simulink model "gg_plus_lc_platoon"  (R2019a)
settings: Solver=ode23t  StartTime=0.0  StopTime=70  FixedStep=0.1  MaxStep=0.01  RelTol=1e-3
InitFcn:
  | load vehStatesBus
libraries: simulink x120, powerlib_meascontrol x14, dspsigops x7, autolibshared x7
(part 5 of 7)

== system gg_plus_lc_platoon/p3/Virtual Vehicle Following ==
  ego : Inport
  virtualLeader : Inport  Port=2
  leaderChange : Inport  Port=3
  extraSpaceFlag : Inport  Port=4
  Enable : EnablePort
  Bus Selector : BusSelector  OutputSignals=X,Xdot,u
  Bus Selector1 : BusSelector  OutputSignals=X,Xdot
  Chart : Stateflow chart  BlockKeywords=__PRM__SERIALIZED__DATA__:Stateflow Chart,Stateflow Diagram  TreatAsAtomicUnit=on
  Compare To Constant : simulink/Logic and Bit Operations/Compare To Constant  relop=>  const=0  OutDataTypeStr=boolean
  Compare To Constant1 : simulink/Logic and Bit Operations/Compare To Constant  relop=<  const=2*maxHeadwayError  OutDataTypeStr=boolean
  Compute Errors : Subsystem
  Mux : Mux  Inputs=2
  Scope : Scope  NumInputPorts=2
  Scope1 : Scope
  Sum : Sum  Inputs=-+|
  Sum6 : Sum  Inputs=|+-
  Terminator : Terminator
  Velocity Control Free Flow : Subsystem  TreatAsAtomicUnit=on
  Velocity Control Min : Subsystem  TreatAsAtomicUnit=on
  Virtual Leader Following : Subsystem  TreatAsAtomicUnit=on
  freeFlowVel : Constant  Value=freeFlowVel
  vMin : Constant  Value=vMin
  u : Outport  InitialOutput=0
  virtualErrors : Outport  Port=2  OutputWhenDisabled=reset  InitialOutput=[0, 0]
  virtualGap : Outport  Port=3  OutputWhenDisabled=reset  InitialOutput=[0]
  vLeaderInRange : Outport  Port=4
  wires:
  leaderChange/1 -> Virtual Leader Following/4(intReset), Compute Errors/6(velFilterReset)
  Compare To Constant1/1 -> Velocity Control Free Flow/3(intReset), vLeaderInRange/1, Chart/2(leaderWithinRange)
  Compare To Constant/1 -> Velocity Control Min/2(intReset)
  Velocity Control Free Flow/1(u) -> Chart/1(uFreeFlowVelControl)
  Sum/1 -> Velocity Control Min/1(ev), Chart/4(velDiff), Compare To Constant/1
  freeFlowVel/1 -> Sum6/1
  Chart/2(u) -> u/1, Scope/2
  Sum6/1 -> Velocity Control Free Flow/1(ev)
  virtualLeader/1 -> Bus Selector1/1
  Mux/1 -> virtualErrors/1
  vMin/1 -> Sum/2
  Compute Errors/1(eh) -> Compare To Constant1/1, Scope1/1, Virtual Leader Following/1(eh), Mux/1
  Bus Selector/3 -> Velocity Control Free Flow/2(realInput), Virtual Leader Following/3(realInput)  "<u>"
  ego/1 -> Bus Selector/1
  Virtual Leader Following/1(u) -> Chart/3(uVehFoll)  "uVehFoll"
  Bus Selector/2 -> Sum6/2, Sum/1, Compute Errors/2(vf)  "<Xdot>"
  Bus Selector/1 -> Compute Errors/1(xf)  "<X>"
  Compute Errors/3("gap ") -> virtualGap/1
  Compute Errors/4(unsafeFlag) -> Terminator/1
  Chart/1(state) -> Scope/1
  Bus Selector1/1 -> Compute Errors/3(xl)  "<X>"
  Velocity Control Min/1(u) -> Chart/5(uMinVelControl)  "uMinVelControl"
  Compute Errors/2(ev) -> Virtual Leader Following/2(ev), Mux/2
  extraSpaceFlag/1 -> Compute Errors/5(extraSpace)
  Bus Selector1/2 -> Compute Errors/4(vl)  "<Xdot>"

== system gg_plus_lc_platoon/p3/controlChoice ==
  state : Inport
  follControl : Inport  Port=2
  leaderInRange : Inport  Port=3
  virtualFollControl : Inport  Port=4
  vLeaderInRange : Inport  Port=5
  ControlChoice : Stateflow chart  BlockKeywords=__PRM__SERIALIZED__DATA__:Stateflow Chart,Stateflow Diagram  TreatAsAtomicUnit=on
  Scope : Scope  NumInputPorts=2
  Scope1 : Scope  NumInputPorts=2
  u : Outport
  wires:
  state/1 -> Scope1/1, ControlChoice/1(state)
  leaderInRange/1 -> Scope1/2, ControlChoice/2(leaderInRange)
  virtualFollControl/1 -> Scope/2, ControlChoice/4(longAdjustmentData)
  follControl/1 -> Scope/1, ControlChoice/3(regVehFollData)
  ControlChoice/1(data) -> u/1  "u"
  vLeaderInRange/1 -> ControlChoice/5(vLeaderInRange)

== system gg_plus_lc_platoon/p3/findLeader ==
  ego : Inport
  all : Inport  Port=2
  lcFlag : Inport  Port=3
  state : Inport  Port=4
  Compare To Constant : simulink/Logic and Bit Operations/Compare To Constant  relop=~=  const=4  OutDataTypeStr=boolean
  NOT : Logic  Operator=NOT  IconShape=distinctive  AllPortsSameDT=off  OutDataTypeStr=boolean
  OR : Logic  Operator=OR  IconShape=distinctive  AllPortsSameDT=off  OutDataTypeStr=boolean
  Selector : Selector  InputPortWidth=8  IndexOptions=Index vector (port)  Indices=[1]  OutputSizes=1
  Subsystem : Subsystem
  Vector Concatenate : Concatenate
  farAwayVeh : Subsystem
  leader : Outport
  leaderIdx : Outport  Port=2  InitialOutput=1
  wires:
  Vector Concatenate/1 -> Selector/1
  farAwayVeh/1(Out1) -> Vector Concatenate/2
  Selector/1 -> leader/1
  NOT/1 -> OR/1
  lcFlag/1 -> NOT/1
  OR/1 -> Subsystem/Enable
  Subsystem/1(idx) -> leaderIdx/1, Selector/2
  all/1 -> Subsystem/2(all), Vector Concatenate/1
  ego/1 -> Subsystem/1(ego), farAwayVeh/1(ego)
  state/1 -> Compare To Constant/1
  Compare To Constant/1 -> OR/2

== system gg_plus_lc_platoon/p3/followerErrors ==
  ego : Inport
  follower : Inport  Port=2
  Bus Selector1 : BusSelector  OutputSignals=X,Xdot
  Bus Selector3 : BusSelector  OutputSignals=X,Xdot
  Mux : Mux  Inputs=2
  Sum3 : Sum  Inputs=-+|
  Terminator1 : Terminator
  gapToFollower : Subsystem
  errors : Outport
  wires:
  gapToFollower/2("gap ") -> Terminator1/1
  Sum3/1 -> Mux/2
  Bus Selector3/2 -> gapToFollower/2(vf), Sum3/1  "<Xdot>"
  follower/1 -> Bus Selector3/1
  gapToFollower/1(eh) -> Mux/1
  Bus Selector1/2 -> Sum3/2  "<Xdot>"
  Bus Selector3/1 -> gapToFollower/1(xf)  "<X>"
  ego/1 -> Bus Selector1/1
  Bus Selector1/1 -> gapToFollower/3(xl)  "<X>"
  Mux/1 -> errors/1

== system gg_plus_lc_platoon/p3/maneuverState ==
  note: States are:
      | 0 - Lane keeping
      | 1 - Longitudinal Adjustment
      | 2 - Steady State
      | 3 - Safe to LC
      | 4 - Performing LC
      | 5 - LC is done
  longAdj : Inport
  steadyState : Inport  Port=2
  safeToVirtualFoll : Inport  Port=3
  canStartLC : Inport  Port=4
  lcDone : Inport  Port=5
  Enable : EnablePort
  AND{,1..3} (4 alike) : Logic  IconShape=distinctive  AllPortsSameDT=off  OutDataTypeStr=fixdt(1,16)
  Data Type Conversion : DataTypeConversion  OutMin=0  OutMax=1  OutDataTypeStr=fixdt(1,16)
  Scope : Scope  NumInputPorts=5
  Sum : Sum  Inputs=+++++
  state : Outport  InitialOutput=0
  wires:
  AND3/1 -> Scope/5, Sum/5
  AND2/1 -> AND3/1, Scope/4, Sum/4
  AND1/1 -> AND2/1, Scope/3, Sum/3
  AND/1 -> AND1/1, Scope/2, Sum/2
  Sum/1 -> state/1
  lcDone/1 -> AND3/2
  canStartLC/1 -> AND2/2
  safeToVirtualFoll/1 -> AND1/2
  steadyState/1 -> AND/2
  longAdj/1 -> Data Type Conversion/1, AND/1
  Data Type Conversion/1 -> Scope/1, Sum/1

== system gg_plus_lc_platoon/p3/safeErrors ==
  errors : Inport
  AND : Logic  IconShape=distinctive  AllPortsSameDT=off  OutDataTypeStr=boolean
  Compare To Constant4 : simulink/Logic and Bit Operations/Compare To Constant  relop=>=  const=-0.1  OutDataTypeStr=boolean
  Demux : Demux  Outputs=2
  Demux1 : Demux  Outputs=2
  Memory : Memory
  Scope : Scope  NumInputPorts=2
  Triggered Subsystem1 : Subsystem  TreatAsAtomicUnit=on
  safetyFlag : Outport
  wires:
  Demux1/2 -> Scope/2
  Demux1/1 -> Scope/1
  Demux/2 -> AND/2
  Demux/1 -> AND/1
  AND/1 -> Triggered Subsystem1/Trigger
  errors/1 -> Compare To Constant4/1, Demux1/1
  Compare To Constant4/1 -> Demux/1
  Triggered Subsystem1/1(Out1) -> Memory/1
  Memory/1 -> safetyFlag/1

== system gg_plus_lc_platoon/p3/virtualVehiclesManager ==
  all : Inport
  longAdj : Inport  Port=2
  lcFlag : Inport  Port=3
  lcDone : Inport  Port=4
  posInPlatoon : Inport  Port=5
  lcStrategy : Inport  Port=6
  Detect Change : simulink/Logic and Bit Operations/Detect Change  vinit=0  OutDataTypeStr=boolean
  MATLAB Function : MATLAB Function  TreatAsAtomicUnit=on
  MATLAB Function1 : MATLAB Function  TreatAsAtomicUnit=on
  Selector : Selector  InputPortWidth=7  IndexOptions=Index vector (port)  Indices=[1]  OutputSizes=1
  Selector1 : Selector  InputPortWidth=7  IndexOptions=Index vector (port)  Indices=[1]  OutputSizes=1
  Width : Width
  virtualVehs : Scope  NumInputPorts=2
  virtualLeader : Outport
  leaderChange : Outport  Port=2
  virtualFollower : Outport  Port=3
  wires:
  Detect Change/1 -> leaderChange/1
  Selector/1 -> virtualLeader/1
  all/1 -> Width/1, Selector1/1, Selector/1
  lcStrategy/1 -> MATLAB Function1/5(lcStrategy), MATLAB Function/6(lcStrategy)
  posInPlatoon/1 -> MATLAB Function1/4(posInPlatoon), MATLAB Function/5(posInPlatoon)
  lcFlag/1 -> MATLAB Function1/3(lcFlag), MATLAB Function/3(lcFlag)
  Width/1 -> MATLAB Function1/1(nVehicles), MATLAB Function/1(nVehicles)
  lcDone/1 -> MATLAB Function/4(lcDone)
  Selector1/1 -> virtualFollower/1
  longAdj/1 -> MATLAB Function1/2(longAdj), MATLAB Function/2(longAdj)
  MATLAB Function/1(virtualLeaderIdx) -> virtualVehs/1, Detect Change/1, Selector/2
  MATLAB Function1/1(virtualFollowerIdx) -> Selector1/2, virtualVehs/2

== system gg_plus_lc_platoon/Fd/Lateral Control/Full State Observer ==
  note: yhat
  note: xhat
  measuredOutputs : Inport
  delta : Inport  Port=2
  Add1 : Sum  Inputs=|-+
  Gain : Gain  Gain=B  Multiplication=Matrix(K*u)
  Gain1 : Gain  Gain=C  Multiplication=Matrix(K*u)
  Gain2 : Gain  Gain=L  Multiplication=Matrix(K*u)
  Gain3 : Gain  Gain=A  Multiplication=Matrix(K*u)
  Integrator : Integrator  InitialCondition=[y0; 0; 0; 0]
  Signal Specification : SignalSpecification  Dimensions=[size(C,1) 1]
  Sum : Sum  Inputs=+++
  xhat : Outport
  wires:
  Gain2/1 -> Sum/1
  Signal Specification/1 -> Gain2/1
  Gain3/1 -> Sum/2
  Gain/1 -> Sum/3
  delta/1 -> Gain/1
  measuredOutputs/1 -> Add1/2
  Sum/1 -> Integrator/1
  Gain1/1 -> Add1/1
  Integrator/1 -> Gain1/1, Gain3/1, xhat/1
  Add1/1 -> Signal Specification/1

== system gg_plus_lc_platoon/Fd/Lateral Control/Triggered Subsystem1 ==
  In1 : Inport
  Trigger : TriggerPort  VariantControl=Variant
  Out1 : Outport  InitialOutput=y0
  wires:
  In1/1 -> Out1/1

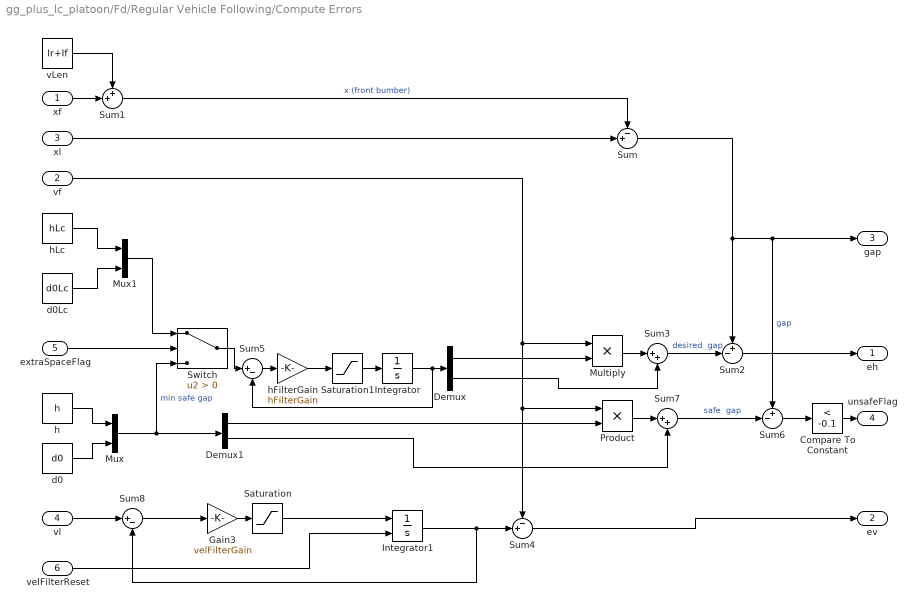
== system gg_plus_lc_platoon/Fd/Regular Vehicle Following/Compute Errors ==
  xf : Inport
  vf : Inport  Port=2
  xl : Inport  Port=3
  vl : Inport  Port=4
  extraSpaceFlag : Inport  Port=5
  velFilterReset : Inport  Port=6
  Compare To Constant : simulink/Logic and Bit Operations/Compare To Constant  relop=<  const=-0.1  OutDataTypeStr=boolean
  Demux : Demux  Outputs=2
  Demux1 : Demux  Outputs=2
  Gain3 : Gain  Gain=velFilterGain
  Integrator : Integrator  InitialCondition=[h d0]
  Integrator1 : Integrator  ExternalReset=rising  InitialCondition=vx0
  Multiply : Product
  Mux : Mux  Inputs=2
  Mux1 : Mux  Inputs=2
  Product : Product
  Saturation : Saturate  UpperLimit=maxAcceleration  LowerLimit=minAcceleration
  Saturation1 : Saturate  UpperLimit=hFilterSaturation  LowerLimit=-hFilterSaturation
  Sum : Sum  Inputs=-+|
  Sum1 : Sum  Inputs=++|
  Sum2 : Sum  Inputs=+-|
  Sum3 : Sum  Inputs=|++
  Sum4 : Sum  Inputs=-+|
  Sum5 : Sum  Inputs=|+-
  Sum6 : Sum  Inputs=+-|
  Sum7 : Sum  Inputs=|++
  Sum8 : Sum  Inputs=|+-
  Switch : Switch  Criteria=u2 > Threshold
  d0 : Constant  Value=d0
  d0Lc : Constant  Value=d0Lc
  h : Constant  Value=h
  hFilterGain : Gain  Gain=hFilterGain
  hLc : Constant  Value=hLc
  vLen : Constant  Value=lr+lf
  eh : Outport
  ev : Outport  Port=2
  "gap " : Outport  Port=3
  unsafeFlag : Outport  Port=4
  wires:
  Sum8/1 -> Gain3/1
  Integrator1/1 -> Sum4/2, Sum8/2
  Saturation/1 -> Integrator1/1
  Gain3/1 -> Saturation/1
  Sum4/1 -> ev/1
  vl/1 -> Sum8/1
  d0Lc/1 -> Mux1/2
  hFilterGain/1 -> Saturation1/1
  Demux/1 -> Multiply/2
  xf/1 -> Sum1/2
  Sum/1 -> Sum2/1, "gap "/1, Sum6/1  "gap"
  Multiply/1 -> Sum3/1
  Demux1/2 -> Sum7/2
  hLc/1 -> Mux1/1
  vLen/1 -> Sum1/1
  Demux/2 -> Sum3/2
  Switch/1 -> Sum5/1
  Sum5/1 -> hFilterGain/1
  vf/1 -> Multiply/1, Product/1, Sum4/1
  Sum1/1 -> Sum/1  "x (front bumber)"
  Sum3/1 -> Sum2/2  "desired  gap"
  h/1 -> Mux/1
  Product/1 -> Sum7/1
  xl/1 -> Sum/2
  extraSpaceFlag/1 -> Switch/2
  Sum2/1 -> eh/1
  Compare To Constant/1 -> unsafeFlag/1
  Demux1/1 -> Product/2
  Integrator/1 -> Sum5/2, Demux/1
  d0/1 -> Mux/2
  Mux1/1 -> Switch/1
  Sum7/1 -> Sum6/2  "safe  gap"
  Mux/1 -> Demux1/1, Switch/3  "min safe gap"
  Sum6/1 -> Compare To Constant/1
  velFilterReset/1 -> Integrator1/2
  Saturation1/1 -> Integrator/1

== system gg_plus_lc_platoon/Fd/Regular Vehicle Following/Veh Following ==
  eh : Inport
  ev : Inport  Port=2
  realInput : Inport  Port=3
  intReset : Inport  Port=4
  Anti-windup gain : Gain  Gain=sqrt(Ki/Kd)
  Integrator : Integrator  ExternalReset=rising
  Kd : Gain  Gain=Kd
  Ki : Gain  Gain=Ki
  Kp : Gain  Gain=Kp
  Saturation1 : Saturate  UpperLimit=maxHeadwayError  LowerLimit=minHeadwayError
  Scope : Scope  NumInputPorts=4
  Sum : Sum  Inputs=|-+
  Sum1 : Sum  Inputs=+++
  Sum5 : Sum  Inputs=-+|
  u : Outport
  wires:
  intReset/1 -> Integrator/2
  ev/1 -> Kd/1
  Ki/1 -> Sum5/2
  Anti-windup gain/1 -> Sum5/1
  Sum5/1 -> Integrator/1
  Kp/1 -> Sum1/2, Scope/2
  Kd/1 -> Sum1/3, Scope/3
  Saturation1/1 -> Ki/1, Kp/1
  eh/1 -> Saturation1/1
  Sum1/1 -> u/1, Sum/2, Scope/4
  realInput/1 -> Sum/1
  Sum/1 -> Anti-windup gain/1
  Integrator/1 -> Scope/1, Sum1/1

== system gg_plus_lc_platoon/Fd/Regular Vehicle Following/Velocity Control ==
  velocity : Inport
  realInput : Inport  Port=2
  intReset : Inport  Port=3
  Anti-windup gain : Gain  Gain=velKp/velKi
  Integrator2 : Integrator  ExternalReset=falling
  Sum : Sum  Inputs=|+-
  Sum1 : Sum  Inputs=|-+
  Sum2 : Sum  Inputs=-+|
  Sum3 : Sum  Inputs=|++
  freeFlowVel : Constant  Value=freeFlowVel
  velKi : Gain  Gain=velKi
  velKp : Gain  Gain=velKp
  u : Outport
  wires:
  Anti-windup gain/1 -> Sum2/1
  Sum/1 -> velKi/1, velKp/1
  velKp/1 -> Sum3/2
  velKi/1 -> Sum2/2
  Integrator2/1 -> Sum3/1
  velocity/1 -> Sum/2
  freeFlowVel/1 -> Sum/1
  intReset/1 -> Integrator2/2
  Sum3/1 -> Sum1/2, u/1
  realInput/1 -> Sum1/1
  Sum1/1 -> Anti-windup gain/1
  Sum2/1 -> Integrator2/1

== system gg_plus_lc_platoon/Fd/Subsystem1/Triggered Subsystem1 ==
  Trigger : TriggerPort  VariantControl=Variant
  Constant : Constant  Value=true  OutDataTypeStr=boolean
  Out1 : Outport  OutDataTypeStr=boolean  InitialOutput=0
  wires:
  Constant/1 -> Out1/1

== system gg_plus_lc_platoon/Fd/Subsystem1/safeErrors1 ==
  errors : Inport
  AND : Logic  IconShape=distinctive  AllPortsSameDT=off  OutDataTypeStr=boolean
  Compare To Constant4 : simulink/Logic and Bit Operations/Compare To Constant  relop=>=  const=-0.1  OutDataTypeStr=boolean
  Demux : Demux  Outputs=2
  safetyFlag : Outport
  wires:
  Compare To Constant4/1 -> Demux/1
  errors/1 -> Compare To Constant4/1
  AND/1 -> safetyFlag/1
  Demux/1 -> AND/1
  Demux/2 -> AND/2

== system gg_plus_lc_platoon/Fd/Subsystem1/safeErrors2 ==
  errors : Inport
  AND : Logic  IconShape=distinctive  AllPortsSameDT=off  OutDataTypeStr=boolean
  Compare To Constant4 : simulink/Logic and Bit Operations/Compare To Constant  relop=>=  const=-0.1  OutDataTypeStr=boolean
  Demux : Demux  Outputs=2
  safetyFlag : Outport
  wires:
  Demux/2 -> AND/2
  Demux/1 -> AND/1
  AND/1 -> safetyFlag/1
  errors/1 -> Compare To Constant4/1
  Compare To Constant4/1 -> Demux/1

== system gg_plus_lc_platoon/Fd/Subsystem1/steadyState ==
  u : Inport
  AND : Logic  IconShape=distinctive  AllPortsSameDT=off  OutDataTypeStr=boolean
  Abs2 : Abs
  Compare To Constant2 : simulink/Logic and Bit Operations/Compare To Constant  relop=<=  const=0.2  OutDataTypeStr=boolean
  Demux : Demux  Outputs=2
  Mux : Mux  Inputs=2
  Transport Delay2 : TransportDelay
  ssFlag : Outport
  wires:
  u/1 -> Transport Delay2/1, Mux/2
  Abs2/1 -> Compare To Constant2/1
  Demux/1 -> AND/1
  Transport Delay2/1 -> Mux/1
  AND/1 -> ssFlag/1
  Compare To Constant2/1 -> Demux/1
  Mux/1 -> Abs2/1
  Demux/2 -> AND/2

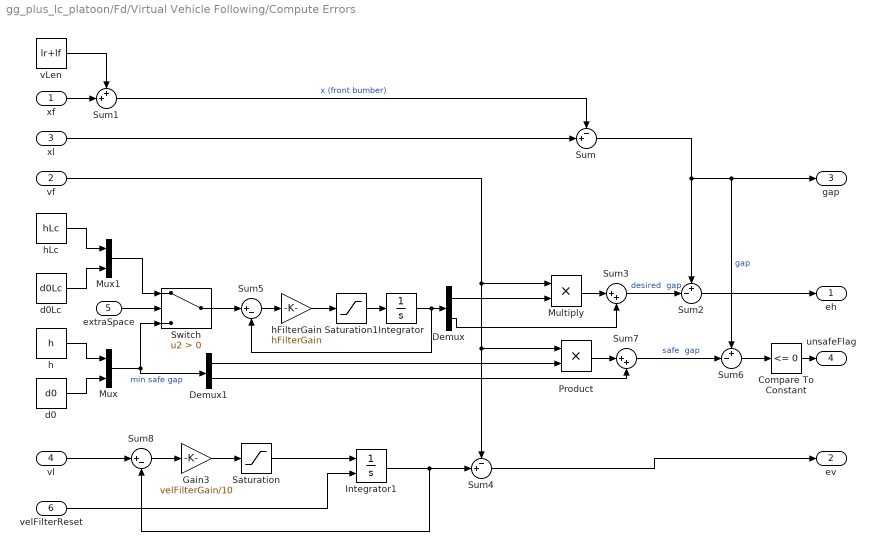
== system gg_plus_lc_platoon/Fd/Virtual Vehicle Following/Compute Errors ==
  xf : Inport
  vf : Inport  Port=2
  xl : Inport  Port=3
  vl : Inport  Port=4
  extraSpace : Inport  Port=5
  velFilterReset : Inport  Port=6
  Compare To Constant : simulink/Logic and Bit Operations/Compare To Constant  relop=<=  const=0  OutDataTypeStr=boolean
  Demux : Demux  Outputs=2
  Demux1 : Demux  Outputs=2
  Gain3 : Gain  Gain=velFilterGain/10
  Integrator : Integrator  InitialCondition=[h d0]
  Integrator1 : Integrator  ExternalReset=rising  InitialCondition=vx0
  Multiply : Product
  Mux : Mux  Inputs=2
  Mux1 : Mux  Inputs=2
  Product : Product
  Saturation : Saturate  UpperLimit=maxAcceleration  LowerLimit=minAcceleration
  Saturation1 : Saturate  UpperLimit=hFilterSaturation  LowerLimit=-hFilterSaturation
  Sum : Sum  Inputs=-+|
  Sum1 : Sum  Inputs=++|
  Sum2 : Sum  Inputs=+-|
  Sum3 : Sum  Inputs=|++
  Sum4 : Sum  Inputs=-+|
  Sum5 : Sum  Inputs=|+-
  Sum6 : Sum  Inputs=+-|
  Sum7 : Sum  Inputs=|++
  Sum8 : Sum  Inputs=|+-
  Switch : Switch  Criteria=u2 > Threshold
  d0 : Constant  Value=d0
  d0Lc : Constant  Value=d0Lc
  h : Constant  Value=h
  hFilterGain : Gain  Gain=hFilterGain
  hLc : Constant  Value=hLc
  vLen : Constant  Value=lr+lf
  eh : Outport
  ev : Outport  Port=2
  "gap " : Outport  Port=3
  unsafeFlag : Outport  Port=4
  wires:
  velFilterReset/1 -> Integrator1/2
  xl/1 -> Sum/2
  Sum6/1 -> Compare To Constant/1
  Mux/1 -> Demux1/1, Switch/3  "min safe gap"
  Sum7/1 -> Sum6/2  "safe  gap"
  Mux1/1 -> Switch/1
  d0/1 -> Mux/2
  Integrator/1 -> Demux/1, Sum5/2
  Demux1/1 -> Product/2
  Compare To Constant/1 -> unsafeFlag/1
  Sum2/1 -> eh/1
  extraSpace/1 -> Switch/2
  Product/1 -> Sum7/1
  h/1 -> Mux/1
  Sum3/1 -> Sum2/2  "desired  gap"
  Sum1/1 -> Sum/1  "x (front bumber)"
  vf/1 -> Sum4/1, Product/1, Multiply/1
  Sum5/1 -> hFilterGain/1
  Switch/1 -> Sum5/1
  Demux/2 -> Sum3/2
  vLen/1 -> Sum1/1
  hLc/1 -> Mux1/1
  Demux1/2 -> Sum7/2
  Multiply/1 -> Sum3/1
  Sum/1 -> Sum6/1, "gap "/1, Sum2/1  "gap"
  xf/1 -> Sum1/2
  Demux/1 -> Multiply/2
  hFilterGain/1 -> Saturation1/1
  d0Lc/1 -> Mux1/2
  Sum4/1 -> ev/1
  Integrator1/1 -> Sum4/2, Sum8/2
  Gain3/1 -> Saturation/1
  Sum8/1 -> Gain3/1
  Saturation/1 -> Integrator1/1
  vl/1 -> Sum8/1
  Saturation1/1 -> Integrator/1

== system gg_plus_lc_platoon/Fd/Virtual Vehicle Following/Velocity Control Free Flow ==
  ev : Inport
  realInput : Inport  Port=2
  intReset : Inport  Port=3
  Anti-windup gain : Gain  Gain=velKp/velKi
  Integrator2 : Integrator  ExternalReset=falling
  Sum1 : Sum  Inputs=|-+
  Sum2 : Sum  Inputs=-+|
  Sum3 : Sum  Inputs=|++
  velKi : Gain  Gain=velKi
  velKp : Gain  Gain=velKp
  u : Outport
  wires:
  Sum2/1 -> Integrator2/1
  Sum1/1 -> Anti-windup gain/1
  realInput/1 -> Sum1/1
  Anti-windup gain/1 -> Sum2/1
  Sum3/1 -> u/1, Sum1/2
  intReset/1 -> Integrator2/2
  Integrator2/1 -> Sum3/1
  velKi/1 -> Sum2/2
  velKp/1 -> Sum3/2
  ev/1 -> velKp/1, velKi/1

== system gg_plus_lc_platoon/Fd/Virtual Vehicle Following/Velocity Control Min ==
  note: Velocity control
  ev : Inport
  intReset : Inport  Port=2
  Integrator2 : Integrator  ExternalReset=rising
  Sum3 : Sum
  velKi : Gain  Gain=velKi
  velKp : Gain  Gain=velKp
  u : Outport
  wires:
  Integrator2/1 -> velKi/1
  velKi/1 -> Sum3/2
  Sum3/1 -> u/1
  velKp/1 -> Sum3/1
  ev/1 -> velKp/1, Integrator2/1
  intReset/1 -> Integrator2/2

== system gg_plus_lc_platoon/Fd/Virtual Vehicle Following/Virtual Leader Following ==
  eh : Inport
  ev : Inport  Port=2
  realInput : Inport  Port=3
  intReset : Inport  Port=4
  Anti-windup gain : Gain  Gain=sqrt(Ki/Kd)
  Gain : Gain  Gain=10
  Integrator : Integrator  ExternalReset=rising
  Integrator2 : Integrator  ExternalReset=rising
  Kd : Gain  Gain=Kd
  Ki : Gain  Gain=Ki
  Kp : Gain  Gain=Kp
  Saturation1 : Saturate  UpperLimit=maxHeadwayError  LowerLimit=minHeadwayError
  Scope : Scope  NumInputPorts=4
  Scope1 : Scope  NumInputPorts=2
  Sum : Sum  Inputs=|-+
  Sum1 : Sum  Inputs=+++
  Sum5 : Sum  Inputs=-+|
  Sum9 : Sum  Inputs=|+-
  u : Outport
  wires:
  Saturation1/1 -> Sum9/1, Scope1/1
  Sum9/1 -> Gain/1
  Gain/1 -> Integrator2/1
  ev/1 -> Kd/1
  Ki/1 -> Sum5/2
  Anti-windup gain/1 -> Sum5/1
  Sum5/1 -> Integrator/1
  Integrator/1 -> Sum1/1, Scope/1
  Kp/1 -> Scope/2, Sum1/2
  Kd/1 -> Scope/3, Sum1/3
  Integrator2/1 -> Kp/1, Ki/1, Scope1/2, Sum9/2
  eh/1 -> Saturation1/1
  Sum1/1 -> Sum/2, u/1, Scope/4
  realInput/1 -> Sum/1
  Sum/1 -> Anti-windup gain/1
  intReset/1 -> Integrator/2, Integrator2/2

== system gg_plus_lc_platoon/Fd/findLeader/Subsystem ==
  ego : Inport
  all : Inport  Port=2
  Enable : EnablePort
  MATLAB Function : MATLAB Function  TreatAsAtomicUnit=on
  idx : Outport  InitialOutput=1
  wires:
  ego/1 -> MATLAB Function/1(ego)
  MATLAB Function/1(leaderIdx) -> idx/1
  all/1 -> MATLAB Function/2(allVehicles)

== system gg_plus_lc_platoon/Fd/findLeader/farAwayVeh ==
  ego : Inport  OutDataTypeStr=Bus: vehStatesBus
  Bus Creator : BusCreator  Inputs=6  OutDataTypeStr=Bus: vehStatesBus  NonVirtualBus=on
  Bus Selector : BusSelector  OutputSignals=X,Y,Xdot,psi,u,delta
  Constant : Constant  Value=1000
  Sum : Sum  Inputs=++|
  Out1 : Outport  OutDataTypeStr=Bus: vehStatesBus
  wires:
  Bus Creator/1 -> Out1/1
  Constant/1 -> Sum/1
  Bus Selector/1 -> Sum/2  "<X>"
  ego/1 -> Bus Selector/1
  Sum/1 -> Bus Creator/1  "X"
  Bus Selector/2 -> Bus Creator/2  "<Y>"
  Bus Selector/3 -> Bus Creator/3  "<Xdot>"
  Bus Selector/4 -> Bus Creator/4  "<psi>"
  Bus Selector/5 -> Bus Creator/5  "<u>"
  Bus Selector/6 -> Bus Creator/6  "<delta>"

== system gg_plus_lc_platoon/Fd/followerErrors/gapToFollower ==
  xf : Inport
  vf : Inport  Port=2
  xl : Inport  Port=3
  Multiply : Product
  Sum : Sum  Inputs=-+|
  Sum1 : Sum  Inputs=++|
  Sum2 : Sum  Inputs=+-|
  Sum3 : Sum  Inputs=|++
  d0 : Constant  Value=d0
  h : Constant  Value=h
  vLen : Constant  Value=lr+lf
  eh : Outport
  "gap " : Outport  Port=2
  wires:
  vLen/1 -> Sum1/1
  Multiply/1 -> Sum3/1
  Sum/1 -> "gap "/1, Sum2/1  "gap"
  xf/1 -> Sum1/2
  Sum3/1 -> Sum2/2  "desired  gap"
  vf/1 -> Multiply/1
  Sum1/1 -> Sum/1  "x (front bumber)"
  xl/1 -> Sum/2
  Sum2/1 -> eh/1
  h/1 -> Multiply/2  "time headway"
  d0/1 -> Sum3/2  "gap at  standstill"

== system gg_plus_lc_platoon/Fd/safeErrors/Triggered Subsystem1 ==
  Trigger : TriggerPort  VariantControl=Variant
  Constant : Constant  Value=true  OutDataTypeStr=boolean
  Out1 : Outport  OutDataTypeStr=boolean  InitialOutput=0
  wires:
  Constant/1 -> Out1/1

== system gg_plus_lc_platoon/Fo/Lateral Control/Full State Observer ==
  note: xhat
  note: yhat
  measuredOutputs : Inport
  delta : Inport  Port=2
  Add1 : Sum  Inputs=|-+
  Gain : Gain  Gain=B  Multiplication=Matrix(K*u)
  Gain1 : Gain  Gain=C  Multiplication=Matrix(K*u)
  Gain2 : Gain  Gain=L  Multiplication=Matrix(K*u)
  Gain3 : Gain  Gain=A  Multiplication=Matrix(K*u)
  Integrator : Integrator  InitialCondition=[y0; 0; 0; 0]
  Signal Specification : SignalSpecification  Dimensions=[size(C,1) 1]
  Sum : Sum  Inputs=+++
  xhat : Outport
  wires:
  Add1/1 -> Signal Specification/1
  Integrator/1 -> xhat/1, Gain3/1, Gain1/1
  Gain1/1 -> Add1/1
  Sum/1 -> Integrator/1
  measuredOutputs/1 -> Add1/2
  delta/1 -> Gain/1
  Gain/1 -> Sum/3
  Gain3/1 -> Sum/2
  Signal Specification/1 -> Gain2/1
  Gain2/1 -> Sum/1

== system gg_plus_lc_platoon/Fo/Lateral Control/Triggered Subsystem1 ==
  In1 : Inport
  Trigger : TriggerPort  VariantControl=Variant
  Out1 : Outport  InitialOutput=y0
  wires:
  In1/1 -> Out1/1

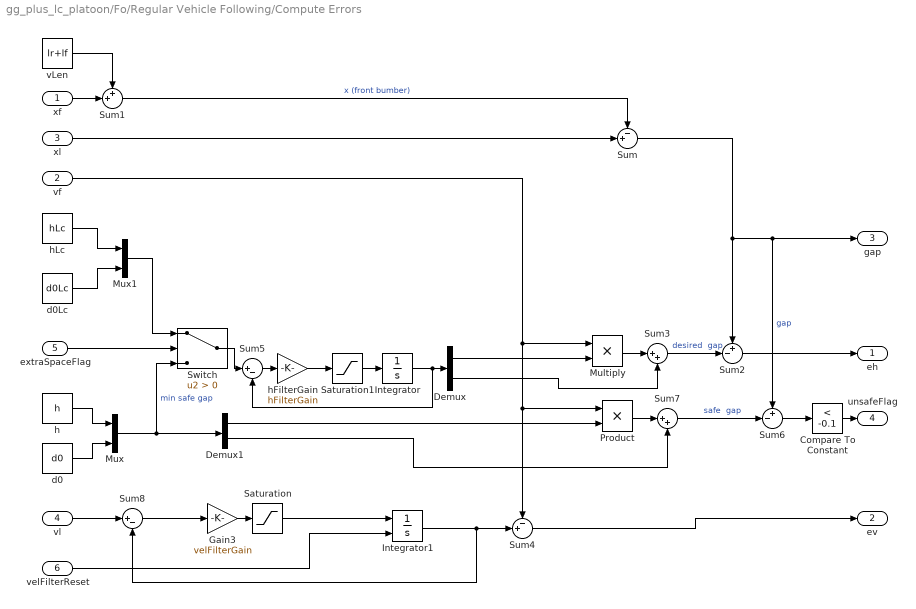
== system gg_plus_lc_platoon/Fo/Regular Vehicle Following/Compute Errors ==
  xf : Inport
  vf : Inport  Port=2
  xl : Inport  Port=3
  vl : Inport  Port=4
  extraSpaceFlag : Inport  Port=5
  velFilterReset : Inport  Port=6
  Compare To Constant : simulink/Logic and Bit Operations/Compare To Constant  relop=<  const=-0.1  OutDataTypeStr=boolean
  Demux : Demux  Outputs=2
  Demux1 : Demux  Outputs=2
  Gain3 : Gain  Gain=velFilterGain
  Integrator : Integrator  InitialCondition=[h d0]
  Integrator1 : Integrator  ExternalReset=rising  InitialCondition=vx0
  Multiply : Product
  Mux : Mux  Inputs=2
  Mux1 : Mux  Inputs=2
  Product : Product
  Saturation : Saturate  UpperLimit=maxAcceleration  LowerLimit=minAcceleration
  Saturation1 : Saturate  UpperLimit=hFilterSaturation  LowerLimit=-hFilterSaturation
  Sum : Sum  Inputs=-+|
  Sum1 : Sum  Inputs=++|
  Sum2 : Sum  Inputs=+-|
  Sum3 : Sum  Inputs=|++
  Sum4 : Sum  Inputs=-+|
  Sum5 : Sum  Inputs=|+-
  Sum6 : Sum  Inputs=+-|
  Sum7 : Sum  Inputs=|++
  Sum8 : Sum  Inputs=|+-
  Switch : Switch  Criteria=u2 > Threshold
  d0 : Constant  Value=d0
  d0Lc : Constant  Value=d0Lc
  h : Constant  Value=h
  hFilterGain : Gain  Gain=hFilterGain
  hLc : Constant  Value=hLc
  vLen : Constant  Value=lr+lf
  eh : Outport
  ev : Outport  Port=2
  "gap " : Outport  Port=3
  unsafeFlag : Outport  Port=4
  wires:
  Saturation1/1 -> Integrator/1
  velFilterReset/1 -> Integrator1/2
  Sum6/1 -> Compare To Constant/1
  Mux/1 -> Switch/3, Demux1/1  "min safe gap"
  Sum7/1 -> Sum6/2  "safe  gap"
  Mux1/1 -> Switch/1
  d0/1 -> Mux/2
  Integrator/1 -> Demux/1, Sum5/2
  Demux1/1 -> Product/2
  Compare To Constant/1 -> unsafeFlag/1
  Sum2/1 -> eh/1
  extraSpaceFlag/1 -> Switch/2
  xl/1 -> Sum/2
  Product/1 -> Sum7/1
  h/1 -> Mux/1
  Sum3/1 -> Sum2/2  "desired  gap"
  Sum1/1 -> Sum/1  "x (front bumber)"
  vf/1 -> Sum4/1, Product/1, Multiply/1
  Sum5/1 -> hFilterGain/1
  Switch/1 -> Sum5/1
  Demux/2 -> Sum3/2
  vLen/1 -> Sum1/1
  hLc/1 -> Mux1/1
  Demux1/2 -> Sum7/2
  Multiply/1 -> Sum3/1
  Sum/1 -> Sum6/1, "gap "/1, Sum2/1  "gap"
  xf/1 -> Sum1/2
  Demux/1 -> Multiply/2
  hFilterGain/1 -> Saturation1/1
  d0Lc/1 -> Mux1/2
  vl/1 -> Sum8/1
  Sum4/1 -> ev/1
  Gain3/1 -> Saturation/1
  Saturation/1 -> Integrator1/1
  Integrator1/1 -> Sum8/2, Sum4/2
  Sum8/1 -> Gain3/1

== system gg_plus_lc_platoon/Fo/Regular Vehicle Following/Veh Following ==
  eh : Inport
  ev : Inport  Port=2
  realInput : Inport  Port=3
  intReset : Inport  Port=4
  Anti-windup gain : Gain  Gain=sqrt(Ki/Kd)
  Integrator : Integrator  ExternalReset=rising
  Kd : Gain  Gain=Kd
  Ki : Gain  Gain=Ki
  Kp : Gain  Gain=Kp
  Saturation1 : Saturate  UpperLimit=maxHeadwayError  LowerLimit=minHeadwayError
  Scope : Scope  NumInputPorts=4
  Sum : Sum  Inputs=|-+
  Sum1 : Sum  Inputs=+++
  Sum5 : Sum  Inputs=-+|
  u : Outport
  wires:
  Integrator/1 -> Sum1/1, Scope/1
  Sum/1 -> Anti-windup gain/1
  realInput/1 -> Sum/1
  Sum1/1 -> Scope/4, Sum/2, u/1
  eh/1 -> Saturation1/1
  Saturation1/1 -> Kp/1, Ki/1
  Kd/1 -> Scope/3, Sum1/3
  Kp/1 -> Scope/2, Sum1/2
  Sum5/1 -> Integrator/1
  Anti-windup gain/1 -> Sum5/1
  Ki/1 -> Sum5/2
  ev/1 -> Kd/1
  intReset/1 -> Integrator/2

== system gg_plus_lc_platoon/Fo/Regular Vehicle Following/Velocity Control ==
  velocity : Inport
  realInput : Inport  Port=2
  intReset : Inport  Port=3
  Anti-windup gain : Gain  Gain=velKp/velKi
  Integrator2 : Integrator  ExternalReset=falling
  Sum : Sum  Inputs=|+-
  Sum1 : Sum  Inputs=|-+
  Sum2 : Sum  Inputs=-+|
  Sum3 : Sum  Inputs=|++
  freeFlowVel : Constant  Value=freeFlowVel
  velKi : Gain  Gain=velKi
  velKp : Gain  Gain=velKp
  u : Outport
  wires:
  Sum2/1 -> Integrator2/1
  Sum1/1 -> Anti-windup gain/1
  realInput/1 -> Sum1/1
  Sum3/1 -> u/1, Sum1/2
  intReset/1 -> Integrator2/2
  freeFlowVel/1 -> Sum/1
  velocity/1 -> Sum/2
  Integrator2/1 -> Sum3/1
  velKi/1 -> Sum2/2
  velKp/1 -> Sum3/2
  Sum/1 -> velKp/1, velKi/1
  Anti-windup gain/1 -> Sum2/1

== system gg_plus_lc_platoon/Fo/Subsystem1/Triggered Subsystem1 ==
  Trigger : TriggerPort  VariantControl=Variant
  Constant : Constant  Value=true  OutDataTypeStr=boolean
  Out1 : Outport  OutDataTypeStr=boolean  InitialOutput=0
  wires:
  Constant/1 -> Out1/1

== system gg_plus_lc_platoon/Fo/Subsystem1/safeErrors1 ==
  errors : Inport
  AND : Logic  IconShape=distinctive  AllPortsSameDT=off  OutDataTypeStr=boolean
  Compare To Constant4 : simulink/Logic and Bit Operations/Compare To Constant  relop=>=  const=-0.1  OutDataTypeStr=boolean
  Demux : Demux  Outputs=2
  safetyFlag : Outport
  wires:
  Demux/2 -> AND/2
  Demux/1 -> AND/1
  AND/1 -> safetyFlag/1
  errors/1 -> Compare To Constant4/1
  Compare To Constant4/1 -> Demux/1

== system gg_plus_lc_platoon/Fo/Subsystem1/safeErrors2 ==
  errors : Inport
  AND : Logic  IconShape=distinctive  AllPortsSameDT=off  OutDataTypeStr=boolean
  Compare To Constant4 : simulink/Logic and Bit Operations/Compare To Constant  relop=>=  const=-0.1  OutDataTypeStr=boolean
  Demux : Demux  Outputs=2
  safetyFlag : Outport
  wires:
  Compare To Constant4/1 -> Demux/1
  errors/1 -> Compare To Constant4/1
  AND/1 -> safetyFlag/1
  Demux/1 -> AND/1
  Demux/2 -> AND/2

== system gg_plus_lc_platoon/Fo/Subsystem1/steadyState ==
  u : Inport
  AND : Logic  IconShape=distinctive  AllPortsSameDT=off  OutDataTypeStr=boolean
  Abs2 : Abs
  Compare To Constant2 : simulink/Logic and Bit Operations/Compare To Constant  relop=<=  const=0.2  OutDataTypeStr=boolean
  Demux : Demux  Outputs=2
  Mux : Mux  Inputs=2
  Transport Delay2 : TransportDelay
  ssFlag : Outport
  wires:
  Demux/2 -> AND/2
  Mux/1 -> Abs2/1
  Compare To Constant2/1 -> Demux/1
  AND/1 -> ssFlag/1
  Transport Delay2/1 -> Mux/1
  Demux/1 -> AND/1
  Abs2/1 -> Compare To Constant2/1
  u/1 -> Mux/2, Transport Delay2/1

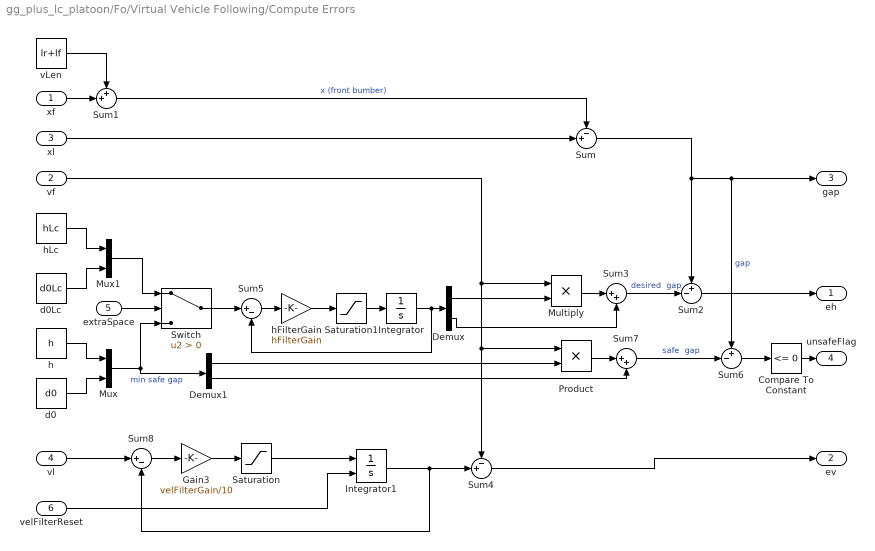
== system gg_plus_lc_platoon/Fo/Virtual Vehicle Following/Compute Errors ==
  xf : Inport
  vf : Inport  Port=2
  xl : Inport  Port=3
  vl : Inport  Port=4
  extraSpace : Inport  Port=5
  velFilterReset : Inport  Port=6
  Compare To Constant : simulink/Logic and Bit Operations/Compare To Constant  relop=<=  const=0  OutDataTypeStr=boolean
  Demux : Demux  Outputs=2
  Demux1 : Demux  Outputs=2
  Gain3 : Gain  Gain=velFilterGain/10
  Integrator : Integrator  InitialCondition=[h d0]
  Integrator1 : Integrator  ExternalReset=rising  InitialCondition=vx0
  Multiply : Product
  Mux : Mux  Inputs=2
  Mux1 : Mux  Inputs=2
  Product : Product
  Saturation : Saturate  UpperLimit=maxAcceleration  LowerLimit=minAcceleration
  Saturation1 : Saturate  UpperLimit=hFilterSaturation  LowerLimit=-hFilterSaturation
  Sum : Sum  Inputs=-+|
  Sum1 : Sum  Inputs=++|
  Sum2 : Sum  Inputs=+-|
  Sum3 : Sum  Inputs=|++
  Sum4 : Sum  Inputs=-+|
  Sum5 : Sum  Inputs=|+-
  Sum6 : Sum  Inputs=+-|
  Sum7 : Sum  Inputs=|++
  Sum8 : Sum  Inputs=|+-
  Switch : Switch  Criteria=u2 > Threshold
  d0 : Constant  Value=d0
  d0Lc : Constant  Value=d0Lc
  h : Constant  Value=h
  hFilterGain : Gain  Gain=hFilterGain
  hLc : Constant  Value=hLc
  vLen : Constant  Value=lr+lf
  eh : Outport
  ev : Outport  Port=2
  "gap " : Outport  Port=3
  unsafeFlag : Outport  Port=4
  wires:
  Saturation1/1 -> Integrator/1
  vl/1 -> Sum8/1
  Saturation/1 -> Integrator1/1
  Sum8/1 -> Gain3/1
  Gain3/1 -> Saturation/1
  Integrator1/1 -> Sum8/2, Sum4/2
  Sum4/1 -> ev/1
  d0Lc/1 -> Mux1/2
  hFilterGain/1 -> Saturation1/1
  Demux/1 -> Multiply/2
  xf/1 -> Sum1/2
  Sum/1 -> Sum2/1, "gap "/1, Sum6/1  "gap"
  Multiply/1 -> Sum3/1
  Demux1/2 -> Sum7/2
  hLc/1 -> Mux1/1
  vLen/1 -> Sum1/1
  Demux/2 -> Sum3/2
  Switch/1 -> Sum5/1
  Sum5/1 -> hFilterGain/1
  vf/1 -> Multiply/1, Product/1, Sum4/1
  Sum1/1 -> Sum/1  "x (front bumber)"
  Sum3/1 -> Sum2/2  "desired  gap"
  h/1 -> Mux/1
  Product/1 -> Sum7/1
  extraSpace/1 -> Switch/2
  Sum2/1 -> eh/1
  Compare To Constant/1 -> unsafeFlag/1
  Demux1/1 -> Product/2
  Integrator/1 -> Sum5/2, Demux/1
  d0/1 -> Mux/2
  Mux1/1 -> Switch/1
  Sum7/1 -> Sum6/2  "safe  gap"
  Mux/1 -> Switch/3, Demux1/1  "min safe gap"
  Sum6/1 -> Compare To Constant/1
  xl/1 -> Sum/2
  velFilterReset/1 -> Integrator1/2

== system gg_plus_lc_platoon/Fo/Virtual Vehicle Following/Velocity Control Free Flow ==
  ev : Inport
  realInput : Inport  Port=2
  intReset : Inport  Port=3
  Anti-windup gain : Gain  Gain=velKp/velKi
  Integrator2 : Integrator  ExternalReset=falling
  Sum1 : Sum  Inputs=|-+
  Sum2 : Sum  Inputs=-+|
  Sum3 : Sum  Inputs=|++
  velKi : Gain  Gain=velKi
  velKp : Gain  Gain=velKp
  u : Outport
  wires:
  ev/1 -> velKi/1, velKp/1
  velKp/1 -> Sum3/2
  velKi/1 -> Sum2/2
  Integrator2/1 -> Sum3/1
  intReset/1 -> Integrator2/2
  Sum3/1 -> Sum1/2, u/1
  Anti-windup gain/1 -> Sum2/1
  realInput/1 -> Sum1/1
  Sum1/1 -> Anti-windup gain/1
  Sum2/1 -> Integrator2/1

== system gg_plus_lc_platoon/Fo/Virtual Vehicle Following/Velocity Control Min ==
  note: Velocity control
  ev : Inport
  intReset : Inport  Port=2
  Integrator2 : Integrator  ExternalReset=rising
  Sum3 : Sum
  velKi : Gain  Gain=velKi
  velKp : Gain  Gain=velKp
  u : Outport
  wires:
  intReset/1 -> Integrator2/2
  ev/1 -> Integrator2/1, velKp/1
  velKp/1 -> Sum3/1
  Sum3/1 -> u/1
  velKi/1 -> Sum3/2
  Integrator2/1 -> velKi/1

== system gg_plus_lc_platoon/Fo/Virtual Vehicle Following/Virtual Leader Following ==
  eh : Inport
  ev : Inport  Port=2
  realInput : Inport  Port=3
  intReset : Inport  Port=4
  Anti-windup gain : Gain  Gain=sqrt(Ki/Kd)
  Gain : Gain  Gain=10
  Integrator : Integrator  ExternalReset=rising
  Integrator2 : Integrator  ExternalReset=rising
  Kd : Gain  Gain=Kd
  Ki : Gain  Gain=Ki
  Kp : Gain  Gain=Kp
  Saturation1 : Saturate  UpperLimit=maxHeadwayError  LowerLimit=minHeadwayError
  Scope : Scope  NumInputPorts=4
  Scope1 : Scope  NumInputPorts=2
  Sum : Sum  Inputs=|-+
  Sum1 : Sum  Inputs=+++
  Sum5 : Sum  Inputs=-+|
  Sum9 : Sum  Inputs=|+-
  u : Outport
  wires:
  intReset/1 -> Integrator2/2, Integrator/2
  Sum/1 -> Anti-windup gain/1
  realInput/1 -> Sum/1
  Sum1/1 -> Scope/4, u/1, Sum/2
  eh/1 -> Saturation1/1
  Integrator2/1 -> Sum9/2, Scope1/2, Ki/1, Kp/1
  Kd/1 -> Sum1/3, Scope/3
  Kp/1 -> Sum1/2, Scope/2
  Integrator/1 -> Scope/1, Sum1/1
  Sum5/1 -> Integrator/1
  Anti-windup gain/1 -> Sum5/1
  Ki/1 -> Sum5/2
  ev/1 -> Kd/1
  Gain/1 -> Integrator2/1
  Sum9/1 -> Gain/1
  Saturation1/1 -> Scope1/1, Sum9/1

== system gg_plus_lc_platoon/Fo/findLeader/Subsystem ==
  ego : Inport
  all : Inport  Port=2
  Enable : EnablePort
  MATLAB Function : MATLAB Function  TreatAsAtomicUnit=on
  idx : Outport  InitialOutput=1
  wires:
  all/1 -> MATLAB Function/2(allVehicles)
  MATLAB Function/1(leaderIdx) -> idx/1
  ego/1 -> MATLAB Function/1(ego)

== system gg_plus_lc_platoon/Fo/findLeader/farAwayVeh ==
  ego : Inport  OutDataTypeStr=Bus: vehStatesBus
  Bus Creator : BusCreator  Inputs=6  OutDataTypeStr=Bus: vehStatesBus  NonVirtualBus=on
  Bus Selector : BusSelector  OutputSignals=X,Y,Xdot,psi,u,delta
  Constant : Constant  Value=1000
  Sum : Sum  Inputs=++|
  Out1 : Outport  OutDataTypeStr=Bus: vehStatesBus
  wires:
  Bus Selector/6 -> Bus Creator/6  "<delta>"
  Bus Selector/5 -> Bus Creator/5  "<u>"
  Bus Selector/4 -> Bus Creator/4  "<psi>"
  Bus Selector/3 -> Bus Creator/3  "<Xdot>"
  Bus Selector/2 -> Bus Creator/2  "<Y>"
  Sum/1 -> Bus Creator/1  "X"
  ego/1 -> Bus Selector/1
  Bus Selector/1 -> Sum/2  "<X>"
  Constant/1 -> Sum/1
  Bus Creator/1 -> Out1/1

== system gg_plus_lc_platoon/Fo/followerErrors/gapToFollower ==
  xf : Inport
  vf : Inport  Port=2
  xl : Inport  Port=3
  Multiply : Product
  Sum : Sum  Inputs=-+|
  Sum1 : Sum  Inputs=++|
  Sum2 : Sum  Inputs=+-|
  Sum3 : Sum  Inputs=|++
  d0 : Constant  Value=d0
  h : Constant  Value=h
  vLen : Constant  Value=lr+lf
  eh : Outport
  "gap " : Outport  Port=2
  wires:
  d0/1 -> Sum3/2  "gap at  standstill"
  h/1 -> Multiply/2  "time headway"
  Sum2/1 -> eh/1
  xl/1 -> Sum/2
  Sum1/1 -> Sum/1  "x (front bumber)"
  vf/1 -> Multiply/1
  Sum3/1 -> Sum2/2  "desired  gap"
  xf/1 -> Sum1/2
  Sum/1 -> Sum2/1, "gap "/1  "gap"
  Multiply/1 -> Sum3/1
  vLen/1 -> Sum1/1

== system gg_plus_lc_platoon/Fo/safeErrors/Triggered Subsystem1 ==
  Trigger : TriggerPort  VariantControl=Variant
  Constant : Constant  Value=true  OutDataTypeStr=boolean
  Out1 : Outport  OutDataTypeStr=boolean  InitialOutput=0
  wires:
  Constant/1 -> Out1/1

== system gg_plus_lc_platoon/Ld/Lateral Control/Full State Observer ==
  note: xhat
  note: yhat
  measuredOutputs : Inport
  delta : Inport  Port=2
  Add1 : Sum  Inputs=|-+
  Gain : Gain  Gain=B  Multiplication=Matrix(K*u)
  Gain1 : Gain  Gain=C  Multiplication=Matrix(K*u)
  Gain2 : Gain  Gain=L  Multiplication=Matrix(K*u)
  Gain3 : Gain  Gain=A  Multiplication=Matrix(K*u)
  Integrator : Integrator  InitialCondition=[y0; 0; 0; 0]
  Signal Specification : SignalSpecification  Dimensions=[size(C,1) 1]
  Sum : Sum  Inputs=+++
  xhat : Outport
  wires:
  Add1/1 -> Signal Specification/1
  Integrator/1 -> xhat/1, Gain3/1, Gain1/1
  Gain1/1 -> Add1/1
  Sum/1 -> Integrator/1
  measuredOutputs/1 -> Add1/2
  delta/1 -> Gain/1
  Gain/1 -> Sum/3
  Gain3/1 -> Sum/2
  Signal Specification/1 -> Gain2/1
  Gain2/1 -> Sum/1

== system gg_plus_lc_platoon/Ld/Lateral Control/Triggered Subsystem1 ==
  In1 : Inport
  Trigger : TriggerPort  VariantControl=Variant
  Out1 : Outport  InitialOutput=y0
  wires:
  In1/1 -> Out1/1

== system gg_plus_lc_platoon/Ld/Regular Vehicle Following/Compute Errors ==
  xf : Inport
  vf : Inport  Port=2
  xl : Inport  Port=3
  vl : Inport  Port=4
  extraSpaceFlag : Inport  Port=5
  velFilterReset : Inport  Port=6
  Compare To Constant : simulink/Logic and Bit Operations/Compare To Constant  relop=<  const=-0.1  OutDataTypeStr=boolean
  Demux : Demux  Outputs=2
  Demux1 : Demux  Outputs=2
  Gain3 : Gain  Gain=velFilterGain
  Integrator : Integrator  InitialCondition=[h d0]
  Integrator1 : Integrator  ExternalReset=rising  InitialCondition=vx0
  Multiply : Product
  Mux : Mux  Inputs=2
  Mux1 : Mux  Inputs=2
  Product : Product
  Saturation : Saturate  UpperLimit=maxAcceleration  LowerLimit=minAcceleration
  Saturation1 : Saturate  UpperLimit=hFilterSaturation  LowerLimit=-hFilterSaturation
  Sum : Sum  Inputs=-+|
  Sum1 : Sum  Inputs=++|
  Sum2 : Sum  Inputs=+-|
  Sum3 : Sum  Inputs=|++
  Sum4 : Sum  Inputs=-+|
  Sum5 : Sum  Inputs=|+-
  Sum6 : Sum  Inputs=+-|
  Sum7 : Sum  Inputs=|++
  Sum8 : Sum  Inputs=|+-
  Switch : Switch  Criteria=u2 > Threshold
  d0 : Constant  Value=d0
  d0Lc : Constant  Value=d0Lc
  h : Constant  Value=h
  hFilterGain : Gain  Gain=hFilterGain
  hLc : Constant  Value=hLc
  vLen : Constant  Value=lr+lf
  eh : Outport
  ev : Outport  Port=2
  "gap " : Outport  Port=3
  unsafeFlag : Outport  Port=4
  wires:
  Saturation1/1 -> Integrator/1
  velFilterReset/1 -> Integrator1/2
  Sum6/1 -> Compare To Constant/1
  Mux/1 -> Switch/3, Demux1/1  "min safe gap"
  Sum7/1 -> Sum6/2  "safe  gap"
  Mux1/1 -> Switch/1
  d0/1 -> Mux/2
  Integrator/1 -> Demux/1, Sum5/2
  Demux1/1 -> Product/2
  Compare To Constant/1 -> unsafeFlag/1
  Sum2/1 -> eh/1
  extraSpaceFlag/1 -> Switch/2
  xl/1 -> Sum/2
  Product/1 -> Sum7/1
  h/1 -> Mux/1
  Sum3/1 -> Sum2/2  "desired  gap"
  Sum1/1 -> Sum/1  "x (front bumber)"
  vf/1 -> Sum4/1, Product/1, Multiply/1
  Sum5/1 -> hFilterGain/1
  Switch/1 -> Sum5/1
  Demux/2 -> Sum3/2
  vLen/1 -> Sum1/1
  hLc/1 -> Mux1/1
  Demux1/2 -> Sum7/2
  Multiply/1 -> Sum3/1
  Sum/1 -> Sum6/1, "gap "/1, Sum2/1  "gap"
  xf/1 -> Sum1/2
  Demux/1 -> Multiply/2
  hFilterGain/1 -> Saturation1/1
  d0Lc/1 -> Mux1/2
  vl/1 -> Sum8/1
  Sum4/1 -> ev/1
  Gain3/1 -> Saturation/1
  Saturation/1 -> Integrator1/1
  Integrator1/1 -> Sum8/2, Sum4/2
  Sum8/1 -> Gain3/1

== system gg_plus_lc_platoon/Ld/Regular Vehicle Following/Veh Following ==
  eh : Inport
  ev : Inport  Port=2
  realInput : Inport  Port=3
  intReset : Inport  Port=4
  Anti-windup gain : Gain  Gain=sqrt(Ki/Kd)
  Integrator : Integrator  ExternalReset=rising
  Kd : Gain  Gain=Kd
  Ki : Gain  Gain=Ki
  Kp : Gain  Gain=Kp
  Saturation1 : Saturate  UpperLimit=maxHeadwayError  LowerLimit=minHeadwayError
  Scope : Scope  NumInputPorts=4
  Sum : Sum  Inputs=|-+
  Sum1 : Sum  Inputs=+++
  Sum5 : Sum  Inputs=-+|
  u : Outport
  wires:
  Integrator/1 -> Sum1/1, Scope/1
  Sum/1 -> Anti-windup gain/1
  realInput/1 -> Sum/1
  Sum1/1 -> Scope/4, Sum/2, u/1
  eh/1 -> Saturation1/1
  Saturation1/1 -> Kp/1, Ki/1
  Kd/1 -> Scope/3, Sum1/3
  Kp/1 -> Scope/2, Sum1/2
  Sum5/1 -> Integrator/1
  Anti-windup gain/1 -> Sum5/1
  Ki/1 -> Sum5/2
  ev/1 -> Kd/1
  intReset/1 -> Integrator/2

== system gg_plus_lc_platoon/Ld/Regular Vehicle Following/Velocity Control ==
  velocity : Inport
  realInput : Inport  Port=2
  intReset : Inport  Port=3
  Anti-windup gain : Gain  Gain=velKp/velKi
  Integrator2 : Integrator  ExternalReset=falling
  Sum : Sum  Inputs=|+-
  Sum1 : Sum  Inputs=|-+
  Sum2 : Sum  Inputs=-+|
  Sum3 : Sum  Inputs=|++
  freeFlowVel : Constant  Value=freeFlowVel
  velKi : Gain  Gain=velKi
  velKp : Gain  Gain=velKp
  u : Outport
  wires:
  Sum2/1 -> Integrator2/1
  Sum1/1 -> Anti-windup gain/1
  realInput/1 -> Sum1/1
  Sum3/1 -> u/1, Sum1/2
  intReset/1 -> Integrator2/2
  freeFlowVel/1 -> Sum/1
  velocity/1 -> Sum/2
  Integrator2/1 -> Sum3/1
  velKi/1 -> Sum2/2
  velKp/1 -> Sum3/2
  Sum/1 -> velKp/1, velKi/1
  Anti-windup gain/1 -> Sum2/1

== system gg_plus_lc_platoon/Ld/Subsystem1/Triggered Subsystem1 ==
  Trigger : TriggerPort  VariantControl=Variant
  Constant : Constant  Value=true  OutDataTypeStr=boolean
  Out1 : Outport  OutDataTypeStr=boolean  InitialOutput=0
  wires:
  Constant/1 -> Out1/1

== system gg_plus_lc_platoon/Ld/Subsystem1/safeErrors1 ==
  errors : Inport
  AND : Logic  IconShape=distinctive  AllPortsSameDT=off  OutDataTypeStr=boolean
  Compare To Constant4 : simulink/Logic and Bit Operations/Compare To Constant  relop=>=  const=-0.1  OutDataTypeStr=boolean
  Demux : Demux  Outputs=2
  safetyFlag : Outport
  wires:
  Demux/2 -> AND/2
  Demux/1 -> AND/1
  AND/1 -> safetyFlag/1
  errors/1 -> Compare To Constant4/1
  Compare To Constant4/1 -> Demux/1

== system gg_plus_lc_platoon/Ld/Subsystem1/safeErrors2 ==
  errors : Inport
  AND : Logic  IconShape=distinctive  AllPortsSameDT=off  OutDataTypeStr=boolean
  Compare To Constant4 : simulink/Logic and Bit Operations/Compare To Constant  relop=>=  const=-0.1  OutDataTypeStr=boolean
  Demux : Demux  Outputs=2
  safetyFlag : Outport
  wires:
  Compare To Constant4/1 -> Demux/1
  errors/1 -> Compare To Constant4/1
  AND/1 -> safetyFlag/1
  Demux/1 -> AND/1
  Demux/2 -> AND/2

== system gg_plus_lc_platoon/Ld/Subsystem1/steadyState ==
  u : Inport
  AND : Logic  IconShape=distinctive  AllPortsSameDT=off  OutDataTypeStr=boolean
  Abs2 : Abs
  Compare To Constant2 : simulink/Logic and Bit Operations/Compare To Constant  relop=<=  const=0.2  OutDataTypeStr=boolean
  Demux : Demux  Outputs=2
  Mux : Mux  Inputs=2
  Transport Delay2 : TransportDelay
  ssFlag : Outport
  wires:
  Demux/2 -> AND/2
  Mux/1 -> Abs2/1
  Compare To Constant2/1 -> Demux/1
  AND/1 -> ssFlag/1
  Transport Delay2/1 -> Mux/1
  Demux/1 -> AND/1
  Abs2/1 -> Compare To Constant2/1
  u/1 -> Mux/2, Transport Delay2/1

== system gg_plus_lc_platoon/Ld/Virtual Vehicle Following/Compute Errors ==
  xf : Inport
  vf : Inport  Port=2
  xl : Inport  Port=3
  vl : Inport  Port=4
  extraSpace : Inport  Port=5
  velFilterReset : Inport  Port=6
  Compare To Constant : simulink/Logic and Bit Operations/Compare To Constant  relop=<=  const=0  OutDataTypeStr=boolean
  Demux : Demux  Outputs=2
  Demux1 : Demux  Outputs=2
  Gain3 : Gain  Gain=velFilterGain/10
  Integrator : Integrator  InitialCondition=[h d0]
  Integrator1 : Integrator  ExternalReset=rising  InitialCondition=vx0
  Multiply : Product
  Mux : Mux  Inputs=2
  Mux1 : Mux  Inputs=2
  Product : Product
  Saturation : Saturate  UpperLimit=maxAcceleration  LowerLimit=minAcceleration
  Saturation1 : Saturate  UpperLimit=hFilterSaturation  LowerLimit=-hFilterSaturation
  Sum : Sum  Inputs=-+|
  Sum1 : Sum  Inputs=++|
  Sum2 : Sum  Inputs=+-|
  Sum3 : Sum  Inputs=|++
  Sum4 : Sum  Inputs=-+|
  Sum5 : Sum  Inputs=|+-
  Sum6 : Sum  Inputs=+-|
  Sum7 : Sum  Inputs=|++
  Sum8 : Sum  Inputs=|+-
  Switch : Switch  Criteria=u2 > Threshold
  d0 : Constant  Value=d0
  d0Lc : Constant  Value=d0Lc
  h : Constant  Value=h
  hFilterGain : Gain  Gain=hFilterGain
  hLc : Constant  Value=hLc
  vLen : Constant  Value=lr+lf
  eh : Outport
  ev : Outport  Port=2
  "gap " : Outport  Port=3
  unsafeFlag : Outport  Port=4
  wires:
  Saturation1/1 -> Integrator/1
  vl/1 -> Sum8/1
  Saturation/1 -> Integrator1/1
  Sum8/1 -> Gain3/1
  Gain3/1 -> Saturation/1
  Integrator1/1 -> Sum8/2, Sum4/2
  Sum4/1 -> ev/1
  d0Lc/1 -> Mux1/2
  hFilterGain/1 -> Saturation1/1
  Demux/1 -> Multiply/2
  xf/1 -> Sum1/2
  Sum/1 -> Sum2/1, "gap "/1, Sum6/1  "gap"
  Multiply/1 -> Sum3/1
  Demux1/2 -> Sum7/2
  hLc/1 -> Mux1/1
  vLen/1 -> Sum1/1
  Demux/2 -> Sum3/2
  Switch/1 -> Sum5/1
  Sum5/1 -> hFilterGain/1
  vf/1 -> Multiply/1, Product/1, Sum4/1
  Sum1/1 -> Sum/1  "x (front bumber)"
  Sum3/1 -> Sum2/2  "desired  gap"
  h/1 -> Mux/1
  Product/1 -> Sum7/1
  extraSpace/1 -> Switch/2
  Sum2/1 -> eh/1
  Compare To Constant/1 -> unsafeFlag/1
  Demux1/1 -> Product/2
  Integrator/1 -> Sum5/2, Demux/1
  d0/1 -> Mux/2
  Mux1/1 -> Switch/1
  Sum7/1 -> Sum6/2  "safe  gap"
  Mux/1 -> Switch/3, Demux1/1  "min safe gap"
  Sum6/1 -> Compare To Constant/1
  xl/1 -> Sum/2
  velFilterReset/1 -> Integrator1/2

== system gg_plus_lc_platoon/Ld/Virtual Vehicle Following/Velocity Control Free Flow ==
  ev : Inport
  realInput : Inport  Port=2
  intReset : Inport  Port=3
  Anti-windup gain : Gain  Gain=velKp/velKi
  Integrator2 : Integrator  ExternalReset=falling
  Sum1 : Sum  Inputs=|-+
  Sum2 : Sum  Inputs=-+|
  Sum3 : Sum  Inputs=|++
  velKi : Gain  Gain=velKi
  velKp : Gain  Gain=velKp
  u : Outport
  wires:
  ev/1 -> velKi/1, velKp/1
  velKp/1 -> Sum3/2
  velKi/1 -> Sum2/2
  Integrator2/1 -> Sum3/1
  intReset/1 -> Integrator2/2
  Sum3/1 -> Sum1/2, u/1
  Anti-windup gain/1 -> Sum2/1
  realInput/1 -> Sum1/1
  Sum1/1 -> Anti-windup gain/1
  Sum2/1 -> Integrator2/1

== system gg_plus_lc_platoon/Ld/Virtual Vehicle Following/Velocity Control Min ==
  note: Velocity control
  ev : Inport
  intReset : Inport  Port=2
  Integrator2 : Integrator  ExternalReset=rising
  Sum3 : Sum
  velKi : Gain  Gain=velKi
  velKp : Gain  Gain=velKp
  u : Outport
  wires:
  intReset/1 -> Integrator2/2
  ev/1 -> Integrator2/1, velKp/1
  velKp/1 -> Sum3/1
  Sum3/1 -> u/1
  velKi/1 -> Sum3/2
  Integrator2/1 -> velKi/1

== system gg_plus_lc_platoon/Ld/Virtual Vehicle Following/Virtual Leader Following ==
  eh : Inport
  ev : Inport  Port=2
  realInput : Inport  Port=3
  intReset : Inport  Port=4
  Anti-windup gain : Gain  Gain=sqrt(Ki/Kd)
  Gain : Gain  Gain=10
  Integrator : Integrator  ExternalReset=rising
  Integrator2 : Integrator  ExternalReset=rising
  Kd : Gain  Gain=Kd
  Ki : Gain  Gain=Ki
  Kp : Gain  Gain=Kp
  Saturation1 : Saturate  UpperLimit=maxHeadwayError  LowerLimit=minHeadwayError
  Scope : Scope  NumInputPorts=4
  Scope1 : Scope  NumInputPorts=2
  Sum : Sum  Inputs=|-+
  Sum1 : Sum  Inputs=+++
  Sum5 : Sum  Inputs=-+|
  Sum9 : Sum  Inputs=|+-
  u : Outport
  wires:
  intReset/1 -> Integrator2/2, Integrator/2
  Sum/1 -> Anti-windup gain/1
  realInput/1 -> Sum/1
  Sum1/1 -> Scope/4, u/1, Sum/2
  eh/1 -> Saturation1/1
  Integrator2/1 -> Sum9/2, Scope1/2, Ki/1, Kp/1
  Kd/1 -> Sum1/3, Scope/3
  Kp/1 -> Sum1/2, Scope/2
  Integrator/1 -> Scope/1, Sum1/1
  Sum5/1 -> Integrator/1
  Anti-windup gain/1 -> Sum5/1
  Ki/1 -> Sum5/2
  ev/1 -> Kd/1
  Gain/1 -> Integrator2/1
  Sum9/1 -> Gain/1
  Saturation1/1 -> Scope1/1, Sum9/1

== system gg_plus_lc_platoon/Ld/findLeader/Subsystem ==
  ego : Inport
  all : Inport  Port=2
  Enable : EnablePort
  MATLAB Function : MATLAB Function  TreatAsAtomicUnit=on
  idx : Outport  InitialOutput=1
  wires:
  all/1 -> MATLAB Function/2(allVehicles)
  MATLAB Function/1(leaderIdx) -> idx/1
  ego/1 -> MATLAB Function/1(ego)

== system gg_plus_lc_platoon/Ld/findLeader/farAwayVeh ==
  ego : Inport  OutDataTypeStr=Bus: vehStatesBus
  Bus Creator : BusCreator  Inputs=6  OutDataTypeStr=Bus: vehStatesBus  NonVirtualBus=on
  Bus Selector : BusSelector  OutputSignals=X,Y,Xdot,psi,u,delta
  Constant : Constant  Value=1000
  Sum : Sum  Inputs=++|
  Out1 : Outport  OutDataTypeStr=Bus: vehStatesBus
  wires:
  Bus Selector/6 -> Bus Creator/6  "<delta>"
  Bus Selector/5 -> Bus Creator/5  "<u>"
  Bus Selector/4 -> Bus Creator/4  "<psi>"
  Bus Selector/3 -> Bus Creator/3  "<Xdot>"
  Bus Selector/2 -> Bus Creator/2  "<Y>"
  Sum/1 -> Bus Creator/1  "X"
  ego/1 -> Bus Selector/1
  Bus Selector/1 -> Sum/2  "<X>"
  Constant/1 -> Sum/1
  Bus Creator/1 -> Out1/1

== system gg_plus_lc_platoon/Ld/followerErrors/gapToFollower ==
  xf : Inport
  vf : Inport  Port=2
  xl : Inport  Port=3
  Multiply : Product
  Sum : Sum  Inputs=-+|
  Sum1 : Sum  Inputs=++|
  Sum2 : Sum  Inputs=+-|
  Sum3 : Sum  Inputs=|++
  d0 : Constant  Value=d0
  h : Constant  Value=h
  vLen : Constant  Value=lr+lf
  eh : Outport
  "gap " : Outport  Port=2
  wires:
  d0/1 -> Sum3/2  "gap at  standstill"
  h/1 -> Multiply/2  "time headway"
  Sum2/1 -> eh/1
  xl/1 -> Sum/2
  Sum1/1 -> Sum/1  "x (front bumber)"
  vf/1 -> Multiply/1
  Sum3/1 -> Sum2/2  "desired  gap"
  xf/1 -> Sum1/2
  Sum/1 -> Sum2/1, "gap "/1  "gap"
  Multiply/1 -> Sum3/1
  vLen/1 -> Sum1/1

== system gg_plus_lc_platoon/Ld/safeErrors/Triggered Subsystem1 ==
  Trigger : TriggerPort  VariantControl=Variant
  Constant : Constant  Value=true  OutDataTypeStr=boolean
  Out1 : Outport  OutDataTypeStr=boolean  InitialOutput=0
  wires:
  Constant/1 -> Out1/1

== system gg_plus_lc_platoon/Lo/Lateral Control/Full State Observer ==
  note: yhat
  note: xhat
  measuredOutputs : Inport
  delta : Inport  Port=2
  Add1 : Sum  Inputs=|-+
  Gain : Gain  Gain=B  Multiplication=Matrix(K*u)
  Gain1 : Gain  Gain=C  Multiplication=Matrix(K*u)
  Gain2 : Gain  Gain=L  Multiplication=Matrix(K*u)
  Gain3 : Gain  Gain=A  Multiplication=Matrix(K*u)
  Integrator : Integrator  InitialCondition=[y0; 0; 0; 0]
  Signal Specification : SignalSpecification  Dimensions=[size(C,1) 1]
  Sum : Sum  Inputs=+++
  xhat : Outport
  wires:
  Gain2/1 -> Sum/1
  Signal Specification/1 -> Gain2/1
  Gain3/1 -> Sum/2
  Gain/1 -> Sum/3
  delta/1 -> Gain/1
  measuredOutputs/1 -> Add1/2
  Sum/1 -> Integrator/1
  Gain1/1 -> Add1/1
  Integrator/1 -> Gain1/1, Gain3/1, xhat/1
  Add1/1 -> Signal Specification/1

== system gg_plus_lc_platoon/Lo/Lateral Control/Triggered Subsystem1 ==
  In1 : Inport
  Trigger : TriggerPort  VariantControl=Variant
  Out1 : Outport  InitialOutput=y0
  wires:
  In1/1 -> Out1/1
